simulink model "PID_Contoller"  (R2020a)
settings: Solver=VariableStepAuto  StartTime=0.0  StopTime=10  RelTol=1e-3
PreLoadFcn:
  | L = 2.75E-6;
  | R = 4;
  | b = 3.5077E-6;
  | J = 3.2284E-6;
  | K = 0.0274;
undefined symbols (not defined in the file or in its folder): Kd, Ki, Kp
settings Model: DataDictionary=Dictionary_Problem4.sldd  Creator=Admin  LastModifiedBy=Admin
settings DataIOCC: SaveOutput=off  SaveTime=off

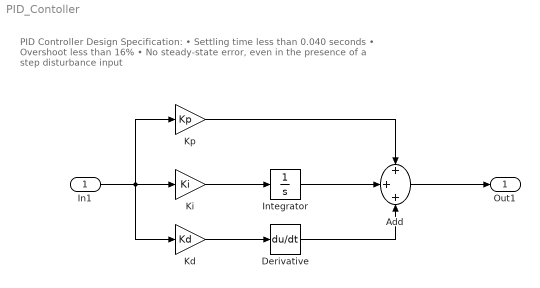
== system PID_Contoller ==
  note: PID Controller Design Specification:
      | • Settling time less than 0.040 seconds
      | • Overshoot less than 16%
      | • No steady-state error, even in the presence of a step disturbance input
  In1 : Inport  OutDataTypeStr=double  PortDimensions=1  SampleTime=0
  Add : Sum  Inputs=+++
  Derivative : Derivative
  Integrator : Integrator
  Kd : Gain  Gain=Kd
  Ki : Gain  Gain=Ki
  Kp : Gain  Gain=Kp
  Out1 : Outport  OutDataTypeStr=double  PortDimensions=1  SampleTime=0
  wires:
  Ki/1 -> Integrator/1
  Derivative/1 -> Add/3
  In1/1 -> Ki/1, Kd/1, Kp/1
  Add/1 -> Out1/1
  Kp/1 -> Add/1
  Integrator/1 -> Add/2
  Kd/1 -> Derivative/1
